simulink library "ECO_TestLibs"  (R2018a)
settings: Solver=ode45  StartTime=0.0  StopTime=10.0  RelTol=1e-3  EnableMultiTasking=on
undefined symbols (not defined in the file or in its folder): h, km
libraries: CoderSF_BSW_Libs x643, $bdroot x217, SF_CanService_Libs x60, simulink x12
(part 1 of 7)
settings Model: Creator=PHS  LastModifiedBy=TianhuaZhang
settings DataIOCC: LimitDataPoints=on  SaveFormat=Array  SignalLoggingSaveFormat=ModelDataLogs
settings OptimizationCC: LifeSpan=inf
settings DebuggingCC: SolverPrmCheckMsg=warning  FcnCallInpInsideContextMsg=warning  SFUnexpectedBacktrackingDiag=warning  SFNoUnconditionalDefaultTransitionDiag=warning  SFExecutionAtInitializationDiag=none
settings HardwareCC: ProdBitPerPointer=32  ProdBitPerSizeT=32  ProdBitPerPtrDiffT=32  ProdLargestAtomicFloat=None  ProdIntDivRoundTo=Undefined  ProdEndianess=Unspecified  ProdWordSize=32  ProdHWDeviceType=32-bit Generic
settings ModelReferenceCC: PropagateSignalLabelsOutOfModel=off
settings CodeAppCC: StateflowObjectComments=on
settings GRTTargetCC: TargetLangStandard=C89/C90 (ANSI)  GeneratePreprocessorConditionals=Disable all  CombineOutputUpdateFcns=off  GRTInterface=on
settings ConfigComp: CovMetricSettings=dw  CovHtmlReporting=on  CovSaveCumulativeToWorkspaceVar=on  CovSaveSingleToWorkspaceVar=on  CovExternalEMLEnable=off

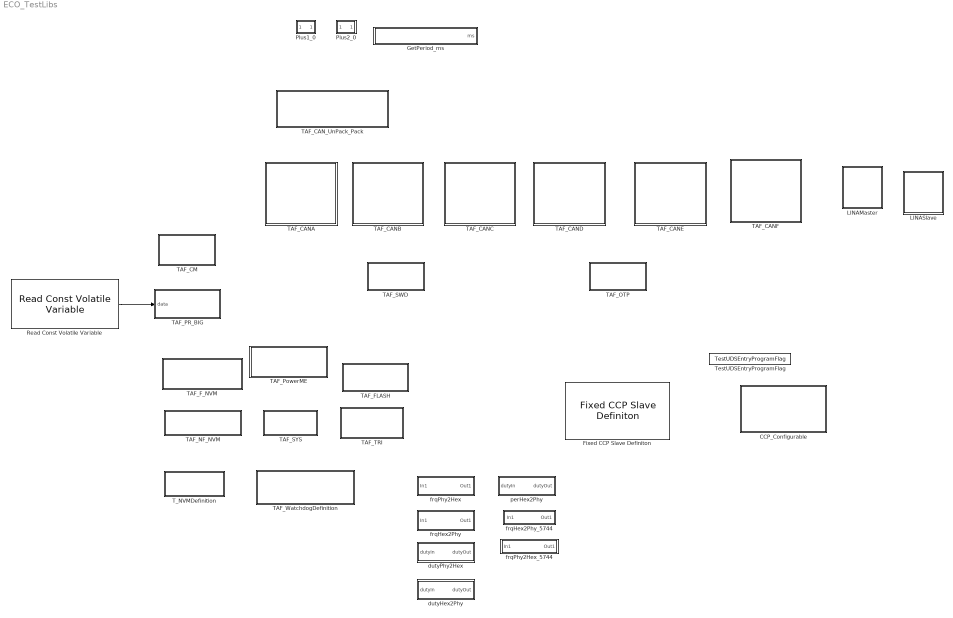
== system ECO_TestLibs ==
  CCP_Configurable : Subsystem
      mask Display: disp('CCP_Configurable');
  Fixed CCP Slave Definiton : CoderSF_BSW_Libs/CCP/Fixed CCP Slave Definiton  ccpType=Simple  ccp_enSet=on  channel=CAN_C  stationaddressSet=hex2dec('0112')  croidSet=hex2dec('100')  dtoidSet=hex2dec('101')  daqidSet=[hex2dec('101') hex2dec('101') hex2dec('101') hex2dec('102')]  daqpidSet=[hex2dec('0') hex2dec('3C') hex2dec('78') hex2dec('0')]  daqlenSet=[hex2dec('0') hex2dec('20') hex2dec('30') hex2dec('30')]  daqperSet=[5 20 100 0]  EcoCoderBlockID=C002_CCPConf
      settings: SourceProductName=EcoCoder Blocks
  GetPeriod_ms : Subsystem  mask{frqP=10000000}
      mask prompts: frqP "Set The Frequence(Hz)"
      mask Display: disp(['The Frequence:',num2str(frqP),'Hz']);
  LINAMaster : Subsystem
  LINASlave : Subsystem
  Plus1_0 : Subsystem  mask(+1){}
      mask help: +1
      mask Display: disp('+1')
  Plus2_0 : Subsystem  mask(+2){}
      mask help: +2
      mask Display: disp('+2')
  Read Const Volatile Variable : CoderSF_BSW_Libs/Variable Blocks/Read Const Volatile Variable  nam='TNF_PRB_DATA'  dataTypeSet=int32  size=2  initialVal=0  dVal=1
      settings: SourceProductName=EcoCoder Blocks
  TAF_CANA : Subsystem
      mask Display: disp('TAF_CANA');
  TAF_CANB : Subsystem
      mask Display: disp('TAF_CANB');
  TAF_CANC : Subsystem
      mask Display: disp('TAF_CANC');
  TAF_CAND : Subsystem
      mask Display: disp('TAF_CAND');
  TAF_CANE : Subsystem
      mask Display: disp('TAF_CANE');
  TAF_CANF : Subsystem
      mask Display: disp('TAF_CANF');
  TAF_CAN_UnPack_Pack : Subsystem
      mask Display: disp('TAF_CAN_UnPack_Pack');
  TAF_CM : Subsystem  mask(numSigle){numSigle=5}
      mask Display: disp('TAF_CM');
  TAF_FLASH : Subsystem
      mask Display: disp('TAF_FLASH');
  TAF_F_NVM : Subsystem  Priority=2
      settings: AttributesFormatString=Priority:%<Priority>
      mask Display: disp('TAF_F_NVM');
  TAF_NF_NVM : Subsystem  Priority=3
      settings: AttributesFormatString=Priority:%<Priority>
      mask Display: disp('TEST_NF_NVM');
  TAF_OTP : Subsystem
      mask Display: disp('TAF_OTP');
  TAF_PR_BIG : Subsystem
      mask Display: disp('TAF_PR_BIG');
  TAF_PowerME : Subsystem  Priority=1
      settings: AttributesFormatString=Priority:%<Priority>
      mask Display: disp('TAF_PowerME');
  TAF_SWD : Subsystem
      mask Display: disp('TAF_SWD');
  TAF_SYS : Subsystem
      mask Display: disp('TAF_SYS');
  TAF_TRI : Subsystem
      mask Display: disp('TAF_TRI');
  TAF_WatchdogDefinition : Subsystem
      mask Display: disp('TAF_WatchdogDefinition');
  T_NVMDefinition : Subsystem
      mask Display: disp('T_NVMDefinition');
  TestUDSEntryProgramFlag : S-Function  FunctionName=TestUDSEntryProgramFlag  SFunctionDeploymentMode=off  EnableBusSupport=off  mask(TestUDSEntryProgramFlag){}
      mask help: TestUDSEntryProgramFlag
  dutyHex2Phy : Subsystem
      mask Display: disp('dutyHex2Phy');
  dutyPhy2Hex : Subsystem
      mask Display: disp('dutyPhy2Hex');
  frqHex2Phy : Subsystem
      mask Display: disp('frqHex2Phy');
  frqHex2Phy_5744 : Subsystem
      mask Display: disp('frqHex2Phy');
  frqPhy2Hex : Subsystem
      mask Display: disp('frqPhy2Hex');
  frqPhy2Hex_5744 : Subsystem
      mask Display: disp('frqPhy2Hex');
  perHex2Phy : Subsystem
      mask Display: disp('perHex2Phy');
  wires:
  Read Const Volatile Variable/1 -> TAF_PR_BIG/1(data)

== system ECO_TestLibs/CCP_Configurable ==
  CCP CAL Seed&Key Security Definiton : CoderSF_BSW_Libs/CCP/CCP CAL Seed&Key Security Definiton  EcoCoderBlockID=CP001_CCPSeedKeyDef  enterloader=on  algorithmEn=on  algorithmTxt=|  keyword1=hex2dec('12')  keyword2=hex2dec('34')  keyword3=hex2dec('56')  keyword4=hex2dec('78')  keyword5=hex2dec('9A')  keyword6=hex2dec('BC')
      | uint8_T i=0;                                 
      |     for(i=0;i<MaxSizeKey;i++)                
      |     {                                        
      |         Key[i]=Seed[i]+1;                    
      |     }                                        
      |     *SizeKey=MaxSizeKey;                     
      |     return 1;
      settings: SourceProductName=EcoCoder Blocks
  CCP DAQ Seed&Key Security Definiton : CoderSF_BSW_Libs/CCP/CCP DAQ Seed&Key Security Definiton  EcoCoderBlockID=CM001_CCPSeedKeyDef  enterloader=on  algorithmEn=on  algorithmTxt=|  keyword1=hex2dec('12')  keyword2=hex2dec('34')  keyword3=hex2dec('56')  keyword4=hex2dec('78')  keyword5=hex2dec('9A')  keyword6=hex2dec('BC')
      | uint8_T i=0;                         
      |     for(i=0;i<MaxSizeKey;i++)        
      |     {                                
      |         Key[i]=Seed[i]+1;            
      |     }                                
      |     *SizeKey=MaxSizeKey;             
      |     return 1;
      settings: SourceProductName=EcoCoder Blocks
  CCP Generate Seed Demo : CoderSF_BSW_Libs/CCP/CCP Generate Seed Demo  facVal=200000
      settings: SourceProductName=EcoCoder Blocks
  CCP PGM Seed&Key Security Definiton : CoderSF_BSW_Libs/CCP/CCP PGM Seed&Key Security Definiton  EcoCoderBlockID=CC001_CCPSeedKeyDef  enterloader=on  algorithmEn=on  algorithmTxt=|  keyword1=hex2dec('12')  keyword2=hex2dec('34')  keyword3=hex2dec('56')  keyword4=hex2dec('78')  keyword5=hex2dec('9A')  keyword6=hex2dec('BC')
      | uint8_T i=0;                                 
      |     for(i=0;i<MaxSizeKey;i++)                
      |     {                                        
      |         Key[i]=Seed[i]+1;                    
      |     }                                        
      |     *SizeKey=MaxSizeKey;                     
      |     return 1;
      settings: SourceProductName=EcoCoder Blocks
  Fixed CCP Slave Definiton : CoderSF_BSW_Libs/CCP/Fixed CCP Slave Definiton  ccpType=Configurable  ccp_enSet=on  channel=CAN_C  stationaddressSet=hex2dec('0112')  croidSet=hex2dec('100')  dtoidSet=hex2dec('101')  daqidSet=[hex2dec('101') hex2dec('101') hex2dec('101') hex2dec('102')]  daqpidSet=[hex2dec('0') hex2dec('3C') hex2dec('78') hex2dec('0')]  daqlenSet=[hex2dec('0') hex2dec('20') hex2dec('30') hex2dec('30')]  daqperSet=[5 20 100 0]  EcoCoderBlockID=C002_CCP21Conf
      settings: SourceProductName=EcoCoder Blocks

== system ECO_TestLibs/GetPeriod_ms ==
  Constant : Constant  Value=frqP  SampleTime=-1
  Constant1 : Constant  Value=1000  OutDataTypeStr=Inherit: Inherit via back propagation  SampleTime=-1
  Divide : Product  Inputs=*/  OutDataTypeStr=single
  Product : Product  OutDataTypeStr=Inherit: Inherit via back propagation
  ReadTBL : CoderSF_BSW_Libs/System Management Blocks/Read System Free Counter
      settings: SourceProductName=EcoCoder Blocks
  Subtract : Sum  Inputs=+-  OutDataTypeStr=Inherit: Same as first input
  Unit Delay : UnitDelay  SampleTime=-1
  ms : Outport
  wires:
  Product/1 -> ms/1
  Subtract/1 -> Divide/1
  ReadTBL/1 -> Subtract/1, Unit Delay/1
  Unit Delay/1 -> Subtract/2
  Constant/1 -> Divide/2
  Divide/1 -> Product/2
  Constant1/1 -> Product/1

== system ECO_TestLibs/LINAMaster ==
  GetStatus : Subsystem
  LIN Channel Definition1 : CoderSF_BSW_Libs/LIN/LIN Channel Definition  EcoCoderBlockID=L001_LINDef  channel=LIN_A  LIN_Mode=LIN_Mode_Master  LIN_Baudrate=9600  Break_Len=13bit
      settings: SourceProductName=EcoCoder Blocks
  RTX : Subsystem
  Task Trigger : CoderSF_BSW_Libs/Task Scheduler/Task Trigger  tasktimeIndex=Task_L100ms
      settings: SourceProductName=EcoCoder Blocks
  Task Trigger1 : CoderSF_BSW_Libs/Task Scheduler/Task Trigger  tasktimeIndex=Task_L10ms
      settings: SourceProductName=EcoCoder Blocks
  wires:
  Task Trigger/1 -> RTX/Trigger
  Task Trigger1/1 -> GetStatus/Trigger
  GetStatus/1(LIN_ST) -> RTX/1(LIN_ST)

== system ECO_TestLibs/LINASlave ==
  LIN Channel Definition : CoderSF_BSW_Libs/LIN/LIN Channel Definition  EcoCoderBlockID=L001_LINDef  channel=LIN_A  LIN_Mode=LIN_Mode_Slave  LIN_Baudrate=9600  Break_Len=13bit
      settings: SourceProductName=EcoCoder Blocks
  Rx : Subsystem  Priority=1
      settings: AttributesFormatString=Priority:%<Priority>
  Task Trigger : CoderSF_BSW_Libs/Task Scheduler/Task Trigger  tasktimeIndex=Task_L100ms
      settings: SourceProductName=EcoCoder Blocks
  Task Trigger1 : CoderSF_BSW_Libs/Task Scheduler/Task Trigger  tasktimeIndex=Task_L100ms
      settings: SourceProductName=EcoCoder Blocks
  Transmit : Subsystem
  wires:
  Task Trigger/1 -> Transmit/Trigger
  Task Trigger1/1 -> Rx/Trigger

== system ECO_TestLibs/Plus1_0 ==
  In1 : Inport
  Add : Sum  OutDataTypeStr=Inherit: Inherit via back propagation
  Constant : Constant  OutDataTypeStr=Inherit: Inherit via back propagation
  Out1 : Outport
  wires:
  Add/1 -> Out1/1
  In1/1 -> Add/1
  Constant/1 -> Add/2

== system ECO_TestLibs/Plus2_0 ==
  In1 : Inport
  Add : Sum  OutDataTypeStr=Inherit: Inherit via back propagation
  Constant : Constant  Value=2  OutDataTypeStr=Inherit: Inherit via back propagation  SampleTime=-1
  Out1 : Outport
  wires:
  Constant/1 -> Add/2
  In1/1 -> Add/1
  Add/1 -> Out1/1

== system ECO_TestLibs/TAF_CANA ==
  CAN Channel Definition : CoderSF_BSW_Libs/CAN/CAN Channel Definition  channel=CAN_A  can_en=on  can_idfilter=off  can_rxextended=on  can_rxMask=hex2dec('0')  can_rxID=hex2dec('200')  can_baudrateIndex=500  can_txbuffer_size=30  can_rxbuffer_size=1  EcoCoderBlockID=C001_CANDef
      settings: SourceProductName=EcoCoder Blocks
  CAN Receive Counter : CoderSF_BSW_Libs/CAN/CAN Receive Counter  channel=CAN_A
      settings: SourceProductName=EcoCoder Blocks
  Connected : Subsystem
  Delay : simulink/Discrete/Integer Delay  NumDelays=1  vinit=0.0  samptime=-1
      settings: SourceProductName=Simulink  SourceProductBaseCode=SL
  Disconnected : Subsystem
  Enabled Subsystem : Subsystem  TreatAsAtomicUnit=on
  Receive CAN Message : Subsystem
  Relational Operator : RelationalOperator  Operator=~=  OutDataTypeStr=boolean  RndMeth=Nearest
  Subsystem : Subsystem
  Write Measurement : CoderSF_BSW_Libs/Calibration & Measurement/Write Measurement  variable_name=TAF_CAN_cntRxA  variable_value=0  variable_type=uint16  numD=1  unitStr=""  descStr=""
      settings: AttributesFormatString=value:%<variable_value> type:%<variable_type>  SourceProductName=EcoCoder Blocks
  wires:
  Delay/1 -> Relational Operator/1
  CAN Receive Counter/1 -> Delay/1, Relational Operator/2, Enabled Subsystem/1(In1), Write Measurement/1
  Relational Operator/1 -> Subsystem/1(In1)
  Subsystem/1(Out1) -> Enabled Subsystem/Enable

== system ECO_TestLibs/TAF_CANB ==
  CAN Channel Definition1 : CoderSF_BSW_Libs/CAN/CAN Channel Definition  channel=CAN_B  can_en=on  can_idfilter=off  can_rxextended=on  can_rxMask=hex2dec('0')  can_rxID=hex2dec('800')  can_baudrateIndex=500  can_txbuffer_size=30  can_rxbuffer_size=1  EcoCoderBlockID=C001_CANDef
      settings: SourceProductName=EcoCoder Blocks
  CAN Receive Counter : CoderSF_BSW_Libs/CAN/CAN Receive Counter  channel=CAN_B
      settings: SourceProductName=EcoCoder Blocks
  Connected : Subsystem
  Delay : simulink/Discrete/Integer Delay  NumDelays=1  vinit=0.0  samptime=-1
      settings: SourceProductName=Simulink  SourceProductBaseCode=SL
  Disconnected : Subsystem
  Enabled Subsystem : Subsystem  TreatAsAtomicUnit=on
  Receive CAN Message : Subsystem
  Relational Operator : RelationalOperator  Operator=~=  OutDataTypeStr=boolean  RndMeth=Nearest
  Subsystem : Subsystem
  Write Measurement : CoderSF_BSW_Libs/Calibration & Measurement/Write Measurement  variable_name=TAF_CAN_cntRxB  variable_value=0  variable_type=uint16  numD=1  unitStr=""  descStr=""
      settings: AttributesFormatString=value:%<variable_value> type:%<variable_type>  SourceProductName=EcoCoder Blocks
  wires:
  Relational Operator/1 -> Subsystem/1(In1)
  Delay/1 -> Relational Operator/1
  CAN Receive Counter/1 -> Delay/1, Relational Operator/2, Enabled Subsystem/1(In1), Write Measurement/1
  Subsystem/1(Out1) -> Enabled Subsystem/Enable

== system ECO_TestLibs/TAF_CANC ==
  CAN Channel Definition2 : CoderSF_BSW_Libs/CAN/CAN Channel Definition  channel=CAN_C  can_en=on  can_idfilter=off  can_rxextended=on  can_rxMask=hex2dec('0')  can_rxID=hex2dec('100')  can_baudrateIndex=500  can_txbuffer_size=30  can_rxbuffer_size=1  EcoCoderBlockID=C001_CANDef
      settings: SourceProductName=EcoCoder Blocks
  CAN Receive Counter2 : CoderSF_BSW_Libs/CAN/CAN Receive Counter  channel=CAN_C
      settings: SourceProductName=EcoCoder Blocks
  Connected : Subsystem
  Delay : simulink/Discrete/Integer Delay  NumDelays=1  vinit=0.0  samptime=-1
      settings: SourceProductName=Simulink  SourceProductBaseCode=SL
  Disconnected : Subsystem
  Enabled Subsystem : Subsystem  TreatAsAtomicUnit=on
  Receive CAN Message : Subsystem
  Relational Operator : RelationalOperator  Operator=~=  OutDataTypeStr=boolean  RndMeth=Nearest
  Subsystem : Subsystem
  Write Measurement2 : CoderSF_BSW_Libs/Calibration & Measurement/Write Measurement  variable_name=TAF_CAN_cntRxC  variable_value=0  variable_type=uint16  numD=1  unitStr=""  descStr=""
      settings: AttributesFormatString=value:%<variable_value> type:%<variable_type>  SourceProductName=EcoCoder Blocks
  wires:
  Delay/1 -> Relational Operator/1
  CAN Receive Counter2/1 -> Delay/1, Relational Operator/2, Enabled Subsystem/1(In1), Write Measurement2/1
  Relational Operator/1 -> Subsystem/1(In1)
  Subsystem/1(Out1) -> Enabled Subsystem/Enable

== system ECO_TestLibs/TAF_CAND ==
  CAN Channel Definition3 : CoderSF_BSW_Libs/CAN/CAN Channel Definition  channel=CAN_D  can_en=on  can_idfilter=off  can_rxextended=on  can_rxMask=hex2dec('0')  can_rxID=hex2dec('100')  can_baudrateIndex=500  can_txbuffer_size=30  can_rxbuffer_size=1  EcoCoderBlockID=C001_CANDef
      settings: SourceProductName=EcoCoder Blocks
  CAN Receive Counter3 : CoderSF_BSW_Libs/CAN/CAN Receive Counter  channel=CAN_D
      settings: SourceProductName=EcoCoder Blocks
  Connected : Subsystem
  Delay : simulink/Discrete/Integer Delay  NumDelays=1  vinit=0.0  samptime=-1
      settings: SourceProductName=Simulink  SourceProductBaseCode=SL
  Disconnected : Subsystem
  Enabled Subsystem : Subsystem  TreatAsAtomicUnit=on
  Receive CAN Message : Subsystem
  Relational Operator : RelationalOperator  Operator=~=  OutDataTypeStr=boolean  RndMeth=Nearest
  Subsystem : Subsystem
  Write Measurement3 : CoderSF_BSW_Libs/Calibration & Measurement/Write Measurement  variable_name=TAF_CAN_cntRxD  variable_value=0  variable_type=uint16  numD=1  unitStr=""  descStr=""
      settings: AttributesFormatString=value:%<variable_value> type:%<variable_type>  SourceProductName=EcoCoder Blocks
  wires:
  Relational Operator/1 -> Subsystem/1(In1)
  Delay/1 -> Relational Operator/1
  CAN Receive Counter3/1 -> Delay/1, Relational Operator/2, Enabled Subsystem/1(In1), Write Measurement3/1
  Subsystem/1(Out1) -> Enabled Subsystem/Enable

== system ECO_TestLibs/TAF_CANE ==
  CAN Channel Definition4 : CoderSF_BSW_Libs/CAN/CAN Channel Definition  channel=CAN_E  can_en=on  can_idfilter=off  can_rxextended=on  can_rxMask=hex2dec('0')  can_rxID=hex2dec('100')  can_baudrateIndex=500  can_txbuffer_size=30  can_rxbuffer_size=1  EcoCoderBlockID=C001_CANDef
      settings: SourceProductName=EcoCoder Blocks
  CAN Receive Counter4 : CoderSF_BSW_Libs/CAN/CAN Receive Counter  channel=CAN_E
      settings: SourceProductName=EcoCoder Blocks
  Connected : Subsystem
  Delay : simulink/Discrete/Integer Delay  NumDelays=1  vinit=0.0  samptime=-1
      settings: SourceProductName=Simulink  SourceProductBaseCode=SL
  Disconnected : Subsystem
  Enabled Subsystem : Subsystem  TreatAsAtomicUnit=on
  Receive CAN Message : Subsystem
  Relational Operator : RelationalOperator  Operator=~=  OutDataTypeStr=boolean  RndMeth=Nearest
  Subsystem : Subsystem
  Write Measurement4 : CoderSF_BSW_Libs/Calibration & Measurement/Write Measurement  variable_name=TAF_CAN_cntRxE  variable_value=0  variable_type=uint16  numD=1  unitStr=""  descStr=""
      settings: AttributesFormatString=value:%<variable_value> type:%<variable_type>  SourceProductName=EcoCoder Blocks
  wires:
  CAN Receive Counter4/1 -> Write Measurement4/1, Enabled Subsystem/1(In1), Relational Operator/2, Delay/1
  Delay/1 -> Relational Operator/1
  Relational Operator/1 -> Subsystem/1(In1)
  Subsystem/1(Out1) -> Enabled Subsystem/Enable

== system ECO_TestLibs/TAF_CANF ==
  CAN Channel Definition4 : CoderSF_BSW_Libs/CAN/CAN Channel Definition  channel=CAN_F  can_en=on  can_idfilter=on  can_rxextended=on  can_rxMask=hex2dec('0')  can_rxID=hex2dec('100')  can_baudrateIndex=500  can_txbuffer_size=30  can_rxbuffer_size=1  EcoCoderBlockID=C001_CANDef
      settings: SourceProductName=EcoCoder Blocks
  CAN Receive Counter4 : CoderSF_BSW_Libs/CAN/CAN Receive Counter  channel=CAN_F
      settings: SourceProductName=EcoCoder Blocks
  Connected : Subsystem
  Delay : simulink/Discrete/Integer Delay  NumDelays=1  vinit=0.0  samptime=-1
      settings: SourceProductName=Simulink  SourceProductBaseCode=SL
  Disconnected : Subsystem
  Enabled Subsystem : Subsystem  TreatAsAtomicUnit=on
  Receive CAN Message : Subsystem
  Relational Operator : RelationalOperator  Operator=~=  OutDataTypeStr=boolean  RndMeth=Nearest
  Subsystem : Subsystem
  Write Measurement4 : CoderSF_BSW_Libs/Calibration & Measurement/Write Measurement  variable_name=TAF_CAN_cntRxF  variable_value=0  variable_type=uint16  numD=1  unitStr=""  descStr=""
      settings: AttributesFormatString=value:%<variable_value> type:%<variable_type>  SourceProductName=EcoCoder Blocks
  wires:
  Relational Operator/1 -> Subsystem/1(In1)
  Delay/1 -> Relational Operator/1
  CAN Receive Counter4/1 -> Delay/1, Relational Operator/2, Enabled Subsystem/1(In1), Write Measurement4/1
  Subsystem/1(Out1) -> Enabled Subsystem/Enable

== system ECO_TestLibs/TAF_CAN_UnPack_Pack ==
  Pack Signals To CAN Data : CoderSF_BSW_Libs/CAN/Pack Signals To CAN Data  Signal="{{'EMS_AcTrq'  'EMS_DmdTrq'},[12 16],[12 12],{'uint16'  'uint16'},{'Motorola' 'Motorola'}}"
      settings: SourceProductName=EcoCoder Blocks
  Read Calibration : CoderSF_BSW_Libs/Calibration & Measurement/Read Calibration  variable_name=TAF_CAN_trqAct_val  variable_value=0  variable_type=uint16  variable_min=[]  variable_max=[]  unitStr=""  descStr=""
      settings: AttributesFormatString=value:%<variable_value> type:%<variable_type> max:%<variable_max> Min:%<variable_min>  SourceProductName=EcoCoder Blocks
  Read Calibration1 : CoderSF_BSW_Libs/Calibration & Measurement/Read Calibration  variable_name=TAF_CAN_trqDmd_val  variable_value=0  variable_type=uint16  variable_min=[]  variable_max=[]  unitStr=""  descStr=""
      settings: AttributesFormatString=value:%<variable_value> type:%<variable_type> max:%<variable_max> Min:%<variable_min>  SourceProductName=EcoCoder Blocks
  Unpack CAN Data To Signals : CoderSF_BSW_Libs/CAN/Unpack CAN Data To Signals  Signal="{{'EMS_AcTrq'  'EMS_DmdTrq'},[12 16],[12 12],{'uint16'  'uint16'},{'Motorola' 'Motorola'}}"
      settings: SourceProductName=EcoCoder Blocks
  Write Measurement : CoderSF_BSW_Libs/Calibration & Measurement/Write Measurement  variable_name=TAF_CAN_trqAct  variable_value=0  variable_type=uint16  numD=1  unitStr=""  descStr=""
      settings: AttributesFormatString=value:%<variable_value> type:%<variable_type>  SourceProductName=EcoCoder Blocks
  Write Measurement1 : CoderSF_BSW_Libs/Calibration & Measurement/Write Measurement  variable_name=TAF_CAN_trqDmd  variable_value=0  variable_type=uint16  numD=1  unitStr=""  descStr=""
      settings: AttributesFormatString=value:%<variable_value> type:%<variable_type>  SourceProductName=EcoCoder Blocks
  wires:
  Read Calibration/1 -> Pack Signals To CAN Data/1
  Read Calibration1/1 -> Pack Signals To CAN Data/2
  Pack Signals To CAN Data/1 -> Unpack CAN Data To Signals/1
  Unpack CAN Data To Signals/2 -> Write Measurement1/1
  Unpack CAN Data To Signals/1 -> Write Measurement/1

== system ECO_TestLibs/TAF_CM ==
  note: 1989
  Calibration Data Check : CoderSF_BSW_Libs/Calibration & Measurement/Calibration Data Check  EcoCoderBlockID=C001_CABCHC  enable_check=on
      settings: SourceProductName=EcoCoder Blocks
  F Calibration Data Check : Subsystem  TreatAsAtomicUnit=on
  Read Calibration : CoderSF_BSW_Libs/Calibration & Measurement/Read Calibration  variable_name=DataRead_flgEn_val  variable_value=0  variable_type=boolean  variable_min=[]  variable_max=[]  unitStr=""  descStr=""
      settings: AttributesFormatString=value:%<variable_value> type:%<variable_type> max:%<variable_max> Min:%<variable_min>  SourceProductName=EcoCoder Blocks
  Read Calibration4 : CoderSF_BSW_Libs/Calibration & Measurement/Read Calibration  variable_name=TCMArray_voltSingle_test  variable_value=zeros(1,numSigle)  variable_type=single  variable_min=[]  variable_max=[]  unitStr=V  descStr=""
      settings: AttributesFormatString=value:%<variable_value> type:%<variable_type> max:%<variable_max> Min:%<variable_min>  SourceProductName=EcoCoder Blocks
  Subsystem : Subsystem
  TAF_DataByAddr : Subsystem
      mask Display: disp('TAF_DataByAddr');
  Write Measurement2 : CoderSF_BSW_Libs/Calibration & Measurement/Write Measurement  variable_name=TCMArray_voltSingle_v  variable_value=0  variable_type=single  numD=numSigle  unitStr=""  descStr=""
      settings: AttributesFormatString=value:%<variable_value> type:%<variable_type>  SourceProductName=EcoCoder Blocks
  wires:
  Calibration Data Check/1 -> F Calibration Data Check/Trigger
  Read Calibration4/1 -> Write Measurement2/1
  Read Calibration/1 -> TAF_DataByAddr/Enable

== system ECO_TestLibs/TAF_FLASH ==
  Online Programming Definition : CoderSF_BSW_Libs/Programming Blocks/Online Programming Definition  EcoCoderBlockID=F001_FlashDef  channel=CAN_A  enable=off  enableOnline=off  cro=hex2dec('100')  dto=hex2dec('101')
      settings: SourceProductName=EcoCoder Blocks
  Online Programming Definition1 : CoderSF_BSW_Libs/Programming Blocks/Online Programming Definition  EcoCoderBlockID=F001_FlashDef  channel=CAN_B  enable=off  enableOnline=off  cro=hex2dec('100')  dto=hex2dec('101')
      settings: SourceProductName=EcoCoder Blocks
  Online Programming Definition2 : CoderSF_BSW_Libs/Programming Blocks/Online Programming Definition  EcoCoderBlockID=F001_FlashDef  channel=CAN_C  enable=on  enableOnline=on  cro=hex2dec('100')  dto=hex2dec('101')
      settings: SourceProductName=EcoCoder Blocks
  Programming SeedKey Definition : CoderSF_BSW_Libs/Programming Blocks/Programming SeedKey Definition  EcoCoderBlockID=S001_SeedKeyDef  enterloader=on  algorithmEn=off  algorithmTxt=|  keyword1=hex2dec('12')  keyword2=hex2dec('34')  keyword3=hex2dec('56')  keyword4=hex2dec('78')  keyword5=hex2dec('9A')  keyword6=hex2dec('BC')
      | uint8_T i=0;
      |     for(i=0;i<MaxSizeKey;i++)
      |     {
      |         Key[i]=2;
      |     }
      |     *SizeKey=MaxSizeKey;    
      |     return 1;
      settings: SourceProductName=EcoCoder Blocks

== system ECO_TestLibs/TAF_F_NVM ==
  FNVM_Read : Subsystem
  FNVM_ReadAndWrite : Subsystem  Priority=2
      settings: AttributesFormatString=%<Priority>
  FNVM_ReadBeforeWrite : Subsystem  Priority=1
      settings: AttributesFormatString=%<Priority>
  Fixed NVM Definition : CoderSF_BSW_Libs/Non-volatile Memory Blocks/Fixed NVM Definition  EcoCoderBlockID=F001_FNVMDef  nvmDefData=ecocoder_getFixedNvmList
      settings: SourceProductName=EcoCoder Blocks
  Task_Call1 : CoderSF_BSW_Libs/Task Scheduler/Task Trigger  tasktimeIndex=Task_L20ms
      settings: SourceProductName=EcoCoder Blocks
  wires:
  Task_Call1/1 -> FNVM_Read/Trigger

== system ECO_TestLibs/TAF_NF_NVM ==
  NVM_Read : Subsystem
  NVM_ReadAndWrite : Subsystem  Priority=2
      settings: AttributesFormatString=%<Priority>
  NVM_ReadBeforeWrite : Subsystem  Priority=1
      settings: AttributesFormatString=%<Priority>
  Task_Call1 : CoderSF_BSW_Libs/Task Scheduler/Task Trigger  tasktimeIndex=Task_L20ms
      settings: SourceProductName=EcoCoder Blocks
  Task_Call4 : CoderSF_BSW_Libs/Task Scheduler/Task Trigger  tasktimeIndex=Task_L5ms
      settings: SourceProductName=EcoCoder Blocks
  Test_NVMStoreFailed : Subsystem  TreatAsAtomicUnit=on
  wires:
  Task_Call4/1 -> Test_NVMStoreFailed/Trigger
  Task_Call1/1 -> NVM_Read/Trigger

== system ECO_TestLibs/TAF_OTP ==
  Calibration Definition : CoderSF_BSW_Libs/Calibration & Measurement/Calibration Definition  variable_name=OTPDiaglog_offset_val  variable_value=3  variable_type=uint32  variable_min=[]  variable_max=[]  unitStr=""  descStr=""
      settings: AttributesFormatString=value:%<variable_value> type:%<variable_type> max:%<variable_max> Min:%<variable_min>  SourceProductName=EcoCoder Blocks
  Calibration Definition1 : CoderSF_BSW_Libs/Calibration & Measurement/Calibration Definition  variable_name=OTPDiaglog_offsetWrite_val  variable_value=2  variable_type=uint32  variable_min=[]  variable_max=[]  unitStr=""  descStr=""
      settings: AttributesFormatString=value:%<variable_value> type:%<variable_type> max:%<variable_max> Min:%<variable_min>  SourceProductName=EcoCoder Blocks
  Read Calibration1 : CoderSF_BSW_Libs/Calibration & Measurement/Read Calibration  variable_name=OTP_offsetRead_val  variable_value=2  variable_type=uint32  variable_min=[]  variable_max=[]  unitStr=""  descStr=""
      settings: AttributesFormatString=value:%<variable_value> type:%<variable_type> max:%<variable_max> Min:%<variable_min>  SourceProductName=EcoCoder Blocks
  Read Calibration2 : CoderSF_BSW_Libs/Calibration & Measurement/Read Calibration  variable_name=OTP_offsetWrite_val  variable_value=2  variable_type=uint32  variable_min=[]  variable_max=[]  unitStr=""  descStr=""
      settings: AttributesFormatString=value:%<variable_value> type:%<variable_type> max:%<variable_max> Min:%<variable_min>  SourceProductName=EcoCoder Blocks
  Read Calibration3 : CoderSF_BSW_Libs/Calibration & Measurement/Read Calibration  variable_name=OTP_dataWrite_val  variable_value=zeros(1,8)  variable_type=uint8  variable_min=[]  variable_max=[]  unitStr=""  descStr=""
      settings: AttributesFormatString=value:%<variable_value> type:%<variable_type> max:%<variable_max> Min:%<variable_min>  SourceProductName=EcoCoder Blocks
  Read Calibration4 : CoderSF_BSW_Libs/Calibration & Measurement/Read Calibration  variable_name=OTP_flgTrigger_val  variable_value=0  variable_type=boolean  variable_min=[]  variable_max=[]  unitStr=""  descStr=""
      settings: AttributesFormatString=value:%<variable_value> type:%<variable_type> max:%<variable_max> Min:%<variable_min>  SourceProductName=EcoCoder Blocks
  Read Calibration6 : CoderSF_BSW_Libs/Calibration & Measurement/Read Calibration  variable_name=OTPDiaglog_dataWrite_val  variable_value=zeros(1,8)  variable_type=uint8  variable_min=[]  variable_max=[]  unitStr=""  descStr=""
      settings: AttributesFormatString=value:%<variable_value> type:%<variable_type> max:%<variable_max> Min:%<variable_min>  SourceProductName=EcoCoder Blocks
  Read Calibration7 : CoderSF_BSW_Libs/Calibration & Measurement/Read Calibration  variable_name=OTPDiaglog_flgTrigger_val  variable_value=0  variable_type=boolean  variable_min=[]  variable_max=[]  unitStr=""  descStr=""
      settings: AttributesFormatString=value:%<variable_value> type:%<variable_type> max:%<variable_max> Min:%<variable_min>  SourceProductName=EcoCoder Blocks
  Read OTP(Input port) : CoderSF_BSW_Libs/Advanced Data Blocks/Read OTP(Input port)  Len=8
      settings: SourceProductName=EcoCoder Blocks
  Read OTP1 : CoderSF_BSW_Libs/Advanced Data Blocks/Read OTP  Len=8  Offset=OTPDiaglog_offset_val
      settings: SourceProductName=EcoCoder Blocks
  Write Measurement1 : CoderSF_BSW_Libs/Calibration & Measurement/Write Measurement  variable_name=OTP_dataRead  variable_value=0  variable_type=uint8  numD=8  unitStr=""  descStr=""
      settings: AttributesFormatString=type:%<variable_type> Dimensions:%<numD>  SourceProductName=EcoCoder Blocks
  Write Measurement2 : CoderSF_BSW_Libs/Calibration & Measurement/Write Measurement  variable_name=OTP_stRead  variable_value=0  variable_type=uint8  numD=1  unitStr=""  descStr=""
      settings: AttributesFormatString=type:%<variable_type> Dimensions:%<numD>  SourceProductName=EcoCoder Blocks
  Write Measurement3 : CoderSF_BSW_Libs/Calibration & Measurement/Write Measurement  variable_name=OTPDiaglog_dataRead  variable_value=0  variable_type=uint8  numD=8  unitStr=""  descStr=""
      settings: AttributesFormatString=type:%<variable_type> Dimensions:%<numD>  SourceProductName=EcoCoder Blocks
  Write Measurement5 : CoderSF_BSW_Libs/Calibration & Measurement/Write Measurement  variable_name=OTPDiaglog_stRead  variable_value=0  variable_type=uint8  numD=1  unitStr=""  descStr=""
      settings: AttributesFormatString=type:%<variable_type> Dimensions:%<numD>  SourceProductName=EcoCoder Blocks
  Write Measurement6 : CoderSF_BSW_Libs/Calibration & Measurement/Write Measurement  variable_name=OTPDiaglog_stWrite  variable_value=0  variable_type=uint8  numD=1  unitStr=""  descStr=""
      settings: AttributesFormatString=type:%<variable_type> Dimensions:%<numD>  SourceProductName=EcoCoder Blocks
  Write Measurement7 : CoderSF_BSW_Libs/Calibration & Measurement/Write Measurement  variable_name=OTP_stWrite  variable_value=0  variable_type=uint8  numD=1  unitStr=""  descStr=""
      settings: AttributesFormatString=type:%<variable_type> Dimensions:%<numD>  SourceProductName=EcoCoder Blocks
  Write OTP(Input port) : CoderSF_BSW_Libs/Advanced Data Blocks/Write OTP(Input port)  TriggerTypeSet=rising  Len=8
      settings: SourceProductName=EcoCoder Blocks
  Write OTP1 : CoderSF_BSW_Libs/Advanced Data Blocks/Write OTP  TriggerTypeSet=rising  Len=8  Offset=OTPDiaglog_offsetWrite_val
      settings: SourceProductName=EcoCoder Blocks
  Write and Read Measurement18 : CoderSF_BSW_Libs/Calibration & Measurement/Write and Read Measurement  variable_name=OTP_flgTrigger  variable_value=0  variable_type=boolean  numD=1  unitStr=""  descStr=""
      settings: AttributesFormatString=type:%<variable_type> Dimensions:%<numD>  SourceProductName=EcoCoder Blocks
  Write and Read Measurement19 : CoderSF_BSW_Libs/Calibration & Measurement/Write and Read Measurement  variable_name=OTPDiaglog_flgTrigger  variable_value=0  variable_type=boolean  numD=1  unitStr=""  descStr=""
      settings: AttributesFormatString=type:%<variable_type> Dimensions:%<numD>  SourceProductName=EcoCoder Blocks
  wires:
  Read OTP1/2 -> Write Measurement5/1
  Read OTP(Input port)/1 -> Write Measurement1/1
  Write OTP(Input port)/1 -> Write Measurement7/1
  Read Calibration4/1 -> Write and Read Measurement18/1
  Read Calibration7/1 -> Write and Read Measurement19/1
  Read OTP1/1 -> Write Measurement3/1
  Write and Read Measurement19/1 -> Write OTP1/Trigger
  Write OTP1/1 -> Write Measurement6/1
  Read OTP(Input port)/2 -> Write Measurement2/1
  Read Calibration6/1 -> Write OTP1/1
  Write and Read Measurement18/1 -> Write OTP(Input port)/Trigger
  Read Calibration1/1 -> Read OTP(Input port)/1
  Read Calibration2/1 -> Write OTP(Input port)/1
  Read Calibration3/1 -> Write OTP(Input port)/2

== system ECO_TestLibs/TAF_PR_BIG ==
  data : Inport
  Data Type Conversion : DataTypeConversion
  Data Type Conversion1 : DataTypeConversion
  Display : Display
  Index Vector : MultiPortSwitch  DataPortOrder=Zero-based contiguous  Inputs=1  zeroidx=on
  Read Calibration1 : CoderSF_BSW_Libs/Calibration & Measurement/Read Calibration  variable_name=PRB_indexData  variable_value=0  variable_type=uint32  variable_min=[]  variable_max=[]  unitStr=""  descStr=""
      settings: AttributesFormatString=value:%<variable_value> type:%<variable_type> max:%<variable_max> Min:%<variable_min>  SourceProductName=EcoCoder Blocks
  Write Measurement1 : CoderSF_BSW_Libs/Calibration & Measurement/Write Measurement  variable_name=PRB_data_single  variable_value=0  variable_type=single  numD=1  unitStr=Nm  descStr=""
      settings: AttributesFormatString=value:%<variable_value> type:%<variable_type>  SourceProductName=EcoCoder Blocks
  Write Measurement2 : CoderSF_BSW_Libs/Calibration & Measurement/Write Measurement  variable_name=PRB_data_int32  variable_value=0  variable_type=int32  numD=1  unitStr=Nm  descStr=""
      settings: AttributesFormatString=value:%<variable_value> type:%<variable_type>  SourceProductName=EcoCoder Blocks
  wires:
  Index Vector/1 -> Data Type Conversion/1, Data Type Conversion1/1
  data/1 -> Index Vector/2
  Read Calibration1/1 -> Index Vector/1
  Data Type Conversion/1 -> Write Measurement1/1, Display/1
  Data Type Conversion1/1 -> Write Measurement2/1

== system ECO_TestLibs/TAF_PowerME ==
  Calibration Definition : CoderSF_BSW_Libs/Calibration & Measurement/Calibration Definition  variable_name=Pwr_tKeyOffDelay_val  variable_value=2.5  variable_type=single  variable_min=[]  variable_max=[]  unitStr=s  descStr=""
      settings: AttributesFormatString=value:%<variable_value> type:%<variable_type> max:%<variable_max> Min:%<variable_min>  SourceProductName=EcoCoder Blocks
  Power Management Example : CoderSF_BSW_Libs/System Management Blocks/Power Management Example  Priority=1  flgKeyFromIn=off  tKeyOffDelaySet=Pwr_tKeyOffDelay_val  flgResetSWEnSet=0  tDbncKeyOffFallSet=0.1  tDbncKeyOffRiseSet=0.1  facAd2VoltSet=109/27846  uKeyOffThrSet=2  uKeyOnHystSet=7  flgCANRxLiveCheckEn=0  flgEnPwrDwnFailReset=1  flgNVMEn=on  tShtDwnWait=500  flgPwrDwnByEdgeTrigger=off  EcoCoderBlockID=PME001_Def
      settings: AttributesFormatString=%<Priority>  SourceProductName=EcoCoder Blocks

== system ECO_TestLibs/TAF_SWD ==
  TAF_SWD : Subsystem
  Task_Call1 : CoderSF_BSW_Libs/Task Scheduler/Task Trigger  tasktimeIndex=Task_L100ms
      settings: SourceProductName=EcoCoder Blocks
  wires:
  Task_Call1/1 -> TAF_SWD/Trigger

== system ECO_TestLibs/TAF_SYS ==
  Function-Call Subsystem1 : Subsystem  TreatAsAtomicUnit=on
  Shutdown Power : Subsystem
  Software Reset : Subsystem
  Task Trigger1 : CoderSF_BSW_Libs/Task Scheduler/Task Trigger  tasktimeIndex=Task_ini
      settings: SourceProductName=EcoCoder Blocks
  wires:
  Task Trigger1/1 -> Function-Call Subsystem1/Trigger

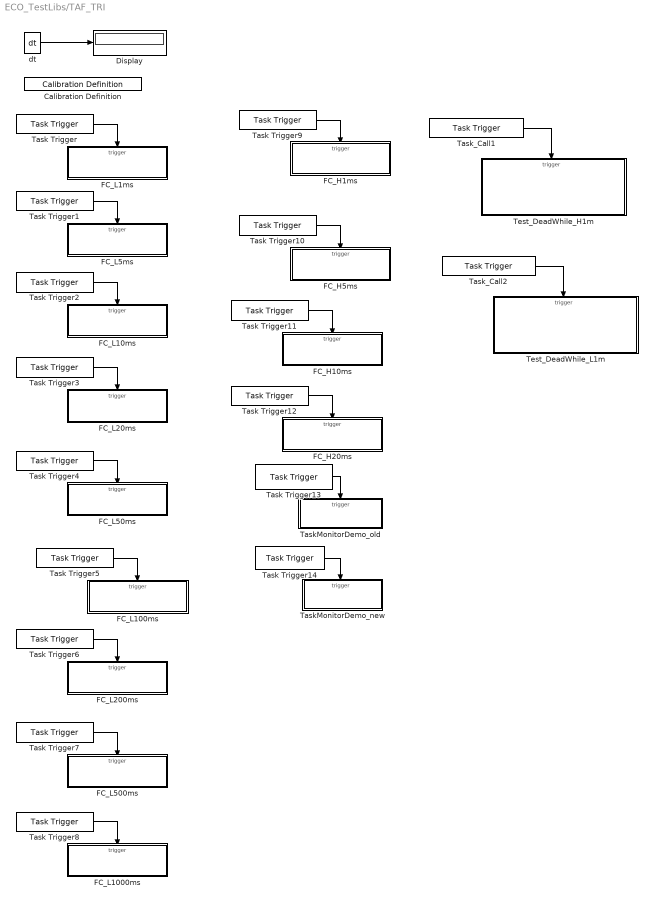
== system ECO_TestLibs/TAF_TRI ==
  Calibration Definition : CoderSF_BSW_Libs/Calibration & Measurement/Calibration Definition  variable_name=TRI_frqFreeSys_val  variable_value=1000  variable_type=single  variable_min=[]  variable_max=[]  unitStr=""  descStr=""
      settings: AttributesFormatString=value:%<variable_value> type:%<variable_type> max:%<variable_max> Min:%<variable_min>  SourceProductName=EcoCoder Blocks
  Display : Display
  FC_H10ms : Subsystem  TreatAsAtomicUnit=on
  FC_H1ms : Subsystem  TreatAsAtomicUnit=on
  FC_H20ms : Subsystem  TreatAsAtomicUnit=on
  FC_H5ms : Subsystem  TreatAsAtomicUnit=on
  FC_L1000ms : Subsystem  TreatAsAtomicUnit=on
  FC_L100ms : Subsystem  TreatAsAtomicUnit=on
  FC_L10ms : Subsystem  TreatAsAtomicUnit=on
  FC_L1ms : Subsystem  TreatAsAtomicUnit=on
  FC_L200ms : Subsystem  TreatAsAtomicUnit=on
  FC_L20ms : Subsystem  TreatAsAtomicUnit=on
  FC_L500ms : Subsystem  TreatAsAtomicUnit=on
  FC_L50ms : Subsystem  TreatAsAtomicUnit=on
  FC_L5ms : Subsystem  TreatAsAtomicUnit=on
  Task Trigger : CoderSF_BSW_Libs/Task Scheduler/Task Trigger  tasktimeIndex=Task_L1ms
      settings: SourceProductName=EcoCoder Blocks
  Task Trigger1 : CoderSF_BSW_Libs/Task Scheduler/Task Trigger  tasktimeIndex=Task_L5ms
      settings: SourceProductName=EcoCoder Blocks
  Task Trigger10 : CoderSF_BSW_Libs/Task Scheduler/Task Trigger  tasktimeIndex=Task_H5ms
      settings: SourceProductName=EcoCoder Blocks
  Task Trigger11 : CoderSF_BSW_Libs/Task Scheduler/Task Trigger  tasktimeIndex=Task_H10ms
      settings: SourceProductName=EcoCoder Blocks
  Task Trigger12 : CoderSF_BSW_Libs/Task Scheduler/Task Trigger  tasktimeIndex=Task_H20ms
      settings: SourceProductName=EcoCoder Blocks
  Task Trigger13 : CoderSF_BSW_Libs/Task Scheduler/Task Trigger  tasktimeIndex=Task_H5ms
      settings: SourceProductName=EcoCoder Blocks
  Task Trigger14 : CoderSF_BSW_Libs/Task Scheduler/Task Trigger  tasktimeIndex=Task_H5ms
      settings: SourceProductName=EcoCoder Blocks
  Task Trigger2 : CoderSF_BSW_Libs/Task Scheduler/Task Trigger  tasktimeIndex=Task_L10ms
      settings: SourceProductName=EcoCoder Blocks
  Task Trigger3 : CoderSF_BSW_Libs/Task Scheduler/Task Trigger  tasktimeIndex=Task_L20ms
      settings: SourceProductName=EcoCoder Blocks
  Task Trigger4 : CoderSF_BSW_Libs/Task Scheduler/Task Trigger  tasktimeIndex=Task_L50ms
      settings: SourceProductName=EcoCoder Blocks
  Task Trigger5 : CoderSF_BSW_Libs/Task Scheduler/Task Trigger  tasktimeIndex=Task_L100ms
      settings: SourceProductName=EcoCoder Blocks
  Task Trigger6 : CoderSF_BSW_Libs/Task Scheduler/Task Trigger  tasktimeIndex=Task_L200ms
      settings: SourceProductName=EcoCoder Blocks
  Task Trigger7 : CoderSF_BSW_Libs/Task Scheduler/Task Trigger  tasktimeIndex=Task_L500ms
      settings: SourceProductName=EcoCoder Blocks
  Task Trigger8 : CoderSF_BSW_Libs/Task Scheduler/Task Trigger  tasktimeIndex=Task_L1000ms
      settings: SourceProductName=EcoCoder Blocks
  Task Trigger9 : CoderSF_BSW_Libs/Task Scheduler/Task Trigger  tasktimeIndex=Task_H1ms
      settings: SourceProductName=EcoCoder Blocks
  TaskMonitorDemo_new : Subsystem
      settings: RTWFcnNameOpts=Use subsystem name
  TaskMonitorDemo_old : Subsystem
      settings: RTWFcnNameOpts=Use subsystem name
  Task_Call1 : CoderSF_BSW_Libs/Task Scheduler/Task Trigger  tasktimeIndex=Task_H1ms
      settings: SourceProductName=EcoCoder Blocks
  Task_Call2 : CoderSF_BSW_Libs/Task Scheduler/Task Trigger  tasktimeIndex=Task_L1ms
      settings: SourceProductName=EcoCoder Blocks
  Test_DeadWhile_H1m : Subsystem  TreatAsAtomicUnit=on
  Test_DeadWhile_L1m : Subsystem  TreatAsAtomicUnit=on
  dt : CoderSF_BSW_Libs/Application Base Blocks/dt
      settings: SourceProductName=EcoCoder Blocks
  wires:
  Task Trigger/1 -> FC_L1ms/Trigger
  Task Trigger1/1 -> FC_L5ms/Trigger
  Task Trigger2/1 -> FC_L10ms/Trigger
  Task Trigger3/1 -> FC_L20ms/Trigger
  Task Trigger4/1 -> FC_L50ms/Trigger
  Task Trigger5/1 -> FC_L100ms/Trigger
  Task Trigger6/1 -> FC_L200ms/Trigger
  Task Trigger7/1 -> FC_L500ms/Trigger
  Task Trigger8/1 -> FC_L1000ms/Trigger
  Task Trigger9/1 -> FC_H1ms/Trigger
  Task Trigger10/1 -> FC_H5ms/Trigger
  Task Trigger11/1 -> FC_H10ms/Trigger
  Task Trigger12/1 -> FC_H20ms/Trigger
  Task_Call1/1 -> Test_DeadWhile_H1m/Trigger
  Task_Call2/1 -> Test_DeadWhile_L1m/Trigger
  Task Trigger13/1 -> TaskMonitorDemo_old/Trigger
  Task Trigger14/1 -> TaskMonitorDemo_new/Trigger
  dt/1 -> Display/1

== system ECO_TestLibs/TAF_WatchdogDefinition ==
  Watchdog  Definition : CoderSF_BSW_Libs/System Management Blocks/Watchdog  Definition  EcoCoderBlockID=W001_WDGConf  soft_en=on  wait_time=500  hard_en=off
      settings: SourceProductName=EcoCoder Blocks

== system ECO_TestLibs/T_NVMDefinition ==
  NVM Definition : CoderSF_BSW_Libs/Non-volatile Memory Blocks/NVM Definition  load=Restore from factory default values in .mot  EcoCoderBlockID=N001_NVMDef
      settings: SourceProductName=EcoCoder Blocks

== system ECO_TestLibs/dutyHex2Phy ==
  dutyIn : Inport
  Product1 : Product  OutDataTypeStr=Inherit: Inherit via back propagation
  Read Calibration1 : CoderSF_BSW_Libs/Calibration & Measurement/Read Calibration  variable_name=TestIPWM_facDuty_val  variable_value=0.01  variable_type=single  variable_min=[]  variable_max=[]  unitStr=""  descStr=""
      settings: AttributesFormatString=value:%<variable_value> type:%<variable_type> max:%<variable_max> Min:%<variable_min>  SourceProductName=EcoCoder Blocks
  dutyOut : Outport
  wires:
  dutyIn/1 -> Product1/1
  Product1/1 -> dutyOut/1
  Read Calibration1/1 -> Product1/2

== system ECO_TestLibs/dutyPhy2Hex ==
  dutyIn : Inport
  Divide : Product  Inputs=*/  OutDataTypeStr=Inherit: Inherit via back propagation
  Read Calibration1 : CoderSF_BSW_Libs/Calibration & Measurement/Read Calibration  variable_name=TestIPWM_facDuty_val  variable_value=0.01  variable_type=single  variable_min=[]  variable_max=[]  unitStr=""  descStr=""
      settings: AttributesFormatString=value:%<variable_value> type:%<variable_type> max:%<variable_max> Min:%<variable_min>  SourceProductName=EcoCoder Blocks
  dutyOut : Outport
  wires:
  Read Calibration1/1 -> Divide/2
  Divide/1 -> dutyOut/1
  dutyIn/1 -> Divide/1

== system ECO_TestLibs/frqHex2Phy ==
  In1 : Inport
  Product : Product  OutDataTypeStr=Inherit: Inherit via back propagation
  Read Calibration : CoderSF_BSW_Libs/Calibration & Measurement/Read Calibration  variable_name=TestIPWM_facFrq_val  variable_value=0.01  variable_type=single  variable_min=[]  variable_max=[]  unitStr=""  descStr=""
      settings: AttributesFormatString=value:%<variable_value> type:%<variable_type> max:%<variable_max> Min:%<variable_min>  SourceProductName=EcoCoder Blocks
  Out1 : Outport
  wires:
  In1/1 -> Product/1
  Read Calibration/1 -> Product/2
  Product/1 -> Out1/1

== system ECO_TestLibs/frqHex2Phy_5744 ==
  In1 : Inport
  Product : Product  OutDataTypeStr=Inherit: Inherit via back propagation
  Read Calibration : CoderSF_BSW_Libs/Calibration & Measurement/Read Calibration  variable_name=TestIPWM_facFrq_val  variable_value=1  variable_type=single  variable_min=[]  variable_max=[]  unitStr=""  descStr=""
      settings: AttributesFormatString=value:%<variable_value> type:%<variable_type> max:%<variable_max> Min:%<variable_min>  SourceProductName=EcoCoder Blocks
  Out1 : Outport
  wires:
  Product/1 -> Out1/1
  Read Calibration/1 -> Product/2
  In1/1 -> Product/1

== system ECO_TestLibs/frqPhy2Hex ==
  In1 : Inport
  Divide : Product  Inputs=*/  OutDataTypeStr=Inherit: Inherit via back propagation
  Read Calibration : CoderSF_BSW_Libs/Calibration & Measurement/Read Calibration  variable_name=TestIPWM_facFrq_val  variable_value=0.01  variable_type=single  variable_min=[]  variable_max=[]  unitStr=""  descStr=""
      settings: AttributesFormatString=value:%<variable_value> type:%<variable_type> max:%<variable_max> Min:%<variable_min>  SourceProductName=EcoCoder Blocks
  Out1 : Outport
  wires:
  Divide/1 -> Out1/1
  Read Calibration/1 -> Divide/2
  In1/1 -> Divide/1

== system ECO_TestLibs/frqPhy2Hex_5744 ==
  In1 : Inport
  Divide : Product  Inputs=*/  OutDataTypeStr=Inherit: Inherit via back propagation
  Read Calibration : CoderSF_BSW_Libs/Calibration & Measurement/Read Calibration  variable_name=TestIPWM_facFrq_val  variable_value=1  variable_type=single  variable_min=[]  variable_max=[]  unitStr=""  descStr=""
      settings: AttributesFormatString=value:%<variable_value> type:%<variable_type> max:%<variable_max> Min:%<variable_min>  SourceProductName=EcoCoder Blocks
  Out1 : Outport
  wires:
  In1/1 -> Divide/1
  Read Calibration/1 -> Divide/2
  Divide/1 -> Out1/1

== system ECO_TestLibs/perHex2Phy ==
  dutyIn : Inport
  Gain : Gain  Gain=0.1  OutDataTypeStr=Inherit: Inherit via back propagation
  dutyOut : Outport
  wires:
  dutyIn/1 -> Gain/1
  Gain/1 -> dutyOut/1

== system ECO_TestLibs/LINAMaster/GetStatus ==
  Trigger : TriggerPort  TriggerType=function-call  VariantControl=(inherit)
  LIN Get Status : CoderSF_BSW_Libs/LIN/LIN Get Status  channel=LIN_A
      settings: SourceProductName=EcoCoder Blocks
  Write and Read Measurement : CoderSF_BSW_Libs/Calibration & Measurement/Write and Read Measurement  variable_name=status  variable_value=0  variable_type=uint8  numD=1  unitStr=""  descStr=""
      settings: AttributesFormatString=type:%<variable_type> Dimensions:%<numD>  SourceProductName=EcoCoder Blocks
  LIN_ST : Outport
  wires:
  LIN Get Status/1 -> Write and Read Measurement/1
  Write and Read Measurement/1 -> LIN_ST/1

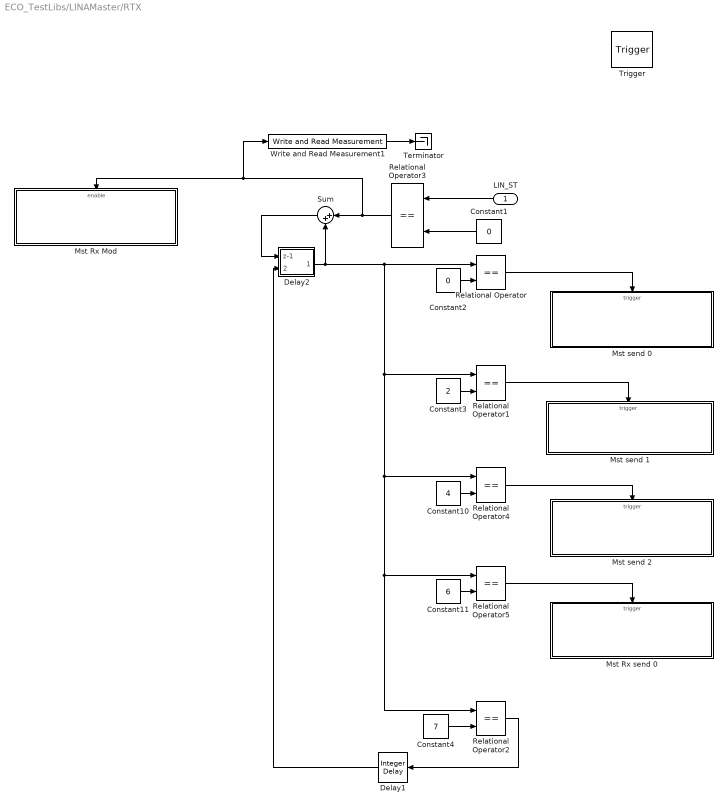
== system ECO_TestLibs/LINAMaster/RTX ==
  LIN_ST : Inport
  Trigger : TriggerPort  TriggerType=function-call  VariantControl=(inherit)
  Constant1 : Constant  Value=0  OutDataTypeStr=uint16
  Constant10 : Constant  Value=4  OutDataTypeStr=uint16
  Constant11 : Constant  Value=6  OutDataTypeStr=uint16
  Constant2 : Constant  Value=0  OutDataTypeStr=uint16
  Constant3 : Constant  Value=2  OutDataTypeStr=uint16
  Constant4 : Constant  Value=7  OutDataTypeStr=uint16
  Delay1 : simulink/Discrete/Integer Delay  NumDelays=1  vinit=0  samptime=-1
      settings: SourceProductName=Simulink  SourceProductBaseCode=SL
  Delay2 : Subsystem
  Mst Rx Mod : Subsystem
      settings: AttributesFormatString=%<Priority>
  Mst Rx send 0 : Subsystem
      settings: AttributesFormatString=%<Priority>
  Mst send 0 : Subsystem
      settings: AttributesFormatString=%<Priority>
  Mst send 1 : Subsystem
      settings: AttributesFormatString=Priority:%<Priority>
  Mst send 2 : Subsystem
      settings: AttributesFormatString=%<Priority>
  Relational Operator{,1..5} (6 alike) : RelationalOperator  Operator===  OutDataTypeStr=boolean  RndMeth=Nearest
  Sum : Sum  Inputs=|++
  Terminator : Terminator
  Write and Read Measurement1 : CoderSF_BSW_Libs/Calibration & Measurement/Write and Read Measurement  variable_name=LIN_BusIdel_Flg  variable_value=0  variable_type=boolean  numD=1  unitStr=""  descStr=""
      settings: AttributesFormatString=type:%<variable_type> Dimensions:%<numD>  SourceProductName=EcoCoder Blocks
  wires:
  Delay2/1(" ") -> Sum/2, Relational Operator4/1, Relational Operator5/1, Relational Operator2/1, Relational Operator1/1, Relational Operator/1
  Sum/1 -> Delay2/1(z-1)
  Constant2/1 -> Relational Operator/2
  Relational Operator/1 -> Mst send 0/Trigger
  Constant3/1 -> Relational Operator1/2
  Relational Operator3/1 -> Write and Read Measurement1/1, Mst Rx Mod/Enable, Sum/1
  Constant4/1 -> Relational Operator2/2
  Relational Operator2/1 -> Delay1/1
  Delay1/1 -> Delay2/2(Rising)
  Constant1/1 -> Relational Operator3/2
  Relational Operator1/1 -> Mst send 1/Trigger
  LIN_ST/1 -> Relational Operator3/1
  Constant10/1 -> Relational Operator4/2
  Relational Operator4/1 -> Mst send 2/Trigger
  Relational Operator5/1 -> Mst Rx send 0/Trigger
  Constant11/1 -> Relational Operator5/2
  Write and Read Measurement1/1 -> Terminator/1

== system ECO_TestLibs/LINASlave/Rx ==
  Trigger : TriggerPort  TriggerType=function-call  VariantControl=(inherit)
  LIN Receive Data3 : CoderSF_BSW_Libs/LIN/LIN Receive Data  channel=LIN_A  Frame_Id=hex2dec('3')  Frame_Len=3  Frame_Dir=MasterSend  Frame_CCS=Classic  Task_TimeIdx=Task_Inherit
      settings: SourceProductName=EcoCoder Blocks
  LIN Receive Data4 : CoderSF_BSW_Libs/LIN/LIN Receive Data  channel=LIN_A  Frame_Id=hex2dec('1')  Frame_Len=3  Frame_Dir=MasterSend  Frame_CCS=Classic  Task_TimeIdx=Task_Inherit
      settings: SourceProductName=EcoCoder Blocks
  LIN Receive Data5 : CoderSF_BSW_Libs/LIN/LIN Receive Data  channel=LIN_A  Frame_Id=hex2dec('2')  Frame_Len=3  Frame_Dir=MasterSend  Frame_CCS=Classic  Task_TimeIdx=Task_Inherit
      settings: SourceProductName=EcoCoder Blocks
  Subsystem : Subsystem
  Subsystem1 : Subsystem
  Subsystem2 : Subsystem
  wires:
  LIN Receive Data3/1 -> Subsystem/Enable
  LIN Receive Data3/2 -> Subsystem/1(In1)
  LIN Receive Data4/2 -> Subsystem1/1(In1)
  LIN Receive Data4/1 -> Subsystem1/Enable
  LIN Receive Data5/2 -> Subsystem2/1(In1)
  LIN Receive Data5/1 -> Subsystem2/Enable

== system ECO_TestLibs/LINASlave/Transmit ==
  Trigger : TriggerPort  TriggerType=function-call  VariantControl=(inherit)
  Tx : Subsystem  Priority=2
      settings: AttributesFormatString=%<Priority>
